simulink model "Position_and_Velocity_Kinematics"  (R2020b)
settings: Solver=VariableStepAuto  StartTime=0.0  StopTime=3  RelTol=1e-3
libraries: simulink x2
settings Model: Creator=barak  LastModifiedBy=barak

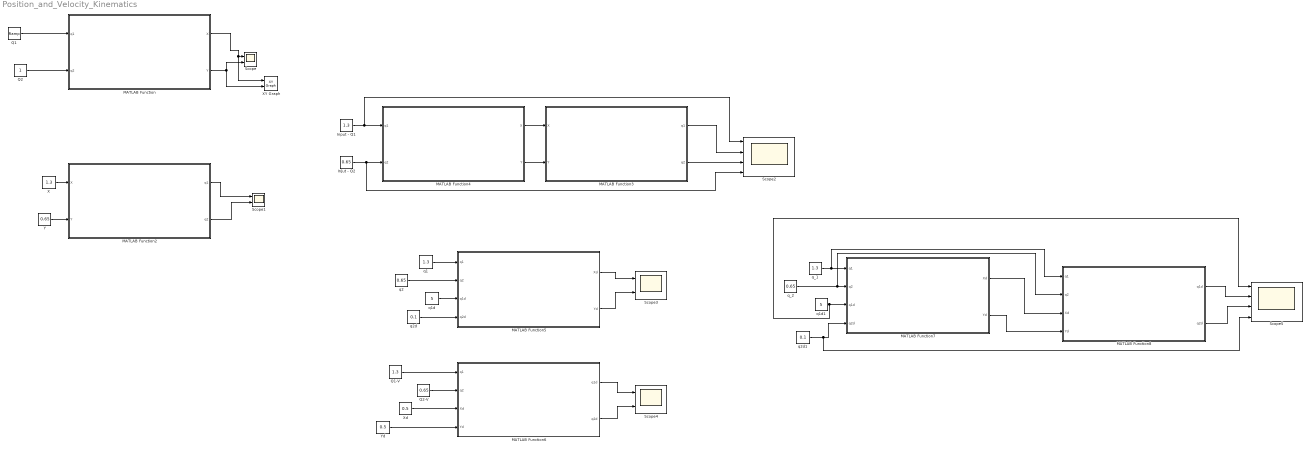
== system Position_and_Velocity_Kinematics ==
  In[ut - Q2 : Constant  Value=0.65
  Input - Q1 : Constant  Value=1.3
  MATLAB Function : MATLAB Function  TreatAsAtomicUnit=on
  MATLAB Function2 : MATLAB Function  TreatAsAtomicUnit=on
  MATLAB Function3 : MATLAB Function  TreatAsAtomicUnit=on
  MATLAB Function4 : MATLAB Function  TreatAsAtomicUnit=on
  MATLAB Function5 : MATLAB Function  TreatAsAtomicUnit=on
  MATLAB Function6 : MATLAB Function  TreatAsAtomicUnit=on
  MATLAB Function7 : MATLAB Function  TreatAsAtomicUnit=on
  MATLAB Function8 : MATLAB Function  TreatAsAtomicUnit=on
  Q1 : simulink/Sources/Ramp  slope=1  start=0  InitialOutput=0
  Q1-V : Constant  Value=1.3
  Q2 : Constant
  Q2-V : Constant  Value=0.65
  Scope{,1,3..4} (4 alike) : Scope  NumInputPorts=2
  Scope2 : Scope  NumInputPorts=4
  Scope5 : Scope  NumInputPorts=4
  X : Constant  Value=1.3
  XY Graph : simulink/Sinks/XY Graph  xmin=-2  xmax=2  ymin=0  ymax=2  st=-1
  Xd : Constant  Value=0.5
  Y : Constant  Value=0.65
  Yd : Constant  Value=0.5
  q1 : Constant  Value=1.3
  q1d : Constant  Value=5
  q1d1 : Constant  Value=5
  q2 : Constant  Value=0.65
  q2d : Constant  Value=0.1
  q2d1 : Constant  Value=0.1
  q_1 : Constant  Value=1.3
  q_2 : Constant  Value=0.65
  wires:
  Q1/1 -> MATLAB Function/1(q1)
  Q2/1 -> MATLAB Function/2(q2)
  MATLAB Function/1(X) -> XY Graph/1, Scope/1
  MATLAB Function/2(Y) -> XY Graph/2, Scope/2
  Y/1 -> MATLAB Function2/2(Y)
  X/1 -> MATLAB Function2/1(X)
  MATLAB Function2/2(q2) -> Scope1/2
  MATLAB Function2/1(q1) -> Scope1/1
  MATLAB Function4/1(X) -> MATLAB Function3/1(X)
  MATLAB Function4/2(Y) -> MATLAB Function3/2(Y)
  In[ut - Q2/1 -> Scope2/4, MATLAB Function4/2(q2)
  Input - Q1/1 -> Scope2/1, MATLAB Function4/1(q1)
  MATLAB Function3/1(q1) -> Scope2/2
  MATLAB Function3/2(q2) -> Scope2/3
  q2/1 -> MATLAB Function5/2(q2)
  q1/1 -> MATLAB Function5/1(q1)
  q1d/1 -> MATLAB Function5/3(q1d)
  q2d/1 -> MATLAB Function5/4(q2d)
  MATLAB Function5/1(Xd) -> Scope3/1
  MATLAB Function5/2(Yd) -> Scope3/2
  Q1-V/1 -> MATLAB Function6/1(q1)
  Q2-V/1 -> MATLAB Function6/2(q2)
  Xd/1 -> MATLAB Function6/3(Xd)
  Yd/1 -> MATLAB Function6/4(Yd)
  MATLAB Function6/2(q2d) -> Scope4/2
  MATLAB Function6/1(q1d) -> Scope4/1
  q2d1/1 -> Scope5/4, MATLAB Function7/4(q2d)
  q_2/1 -> MATLAB Function8/2(q2), MATLAB Function7/2(q2)
  q1d1/1 -> MATLAB Function7/3(q1d), Scope5/1
  q_1/1 -> MATLAB Function8/1(q1), MATLAB Function7/1(q1)
  MATLAB Function7/1(Xd) -> MATLAB Function8/3(Xd)
  MATLAB Function7/2(Yd) -> MATLAB Function8/4(Yd)
  MATLAB Function8/1(q1d) -> Scope5/2
  MATLAB Function8/2(q2d) -> Scope5/3

== matlab function Position_and_Velocity_Kinematics/MATLAB Function ==
  data: q1 input; q2 input; X output; Y output
function [X,Y] = RP_POSITION_FW(q1,q2)
L1 = 0.5;
X = (L1+q2) * cosd(q1);
Y = (L1+q2) * sind(q1);
end

== matlab function Position_and_Velocity_Kinematics/MATLAB Function2 ==
  data: X input; Y input; q1 output; q2 output
function [q1,q2] = RP_POSITION_INV(X,Y)
L1 = 0.5;
q1 = atand(Y/X);
q2 = sqrt(X^2 + Y^2) - L1;
end

== matlab function Position_and_Velocity_Kinematics/MATLAB Function3 ==
  data: X input; Y input; q1 output; q2 output
function [q1,q2] = RP_POSITION_INV(X,Y)
L1 = 0.5;
q1 = atand(Y/X);
q2 = sqrt(X^2 + Y^2) - L1;
end

== matlab function Position_and_Velocity_Kinematics/MATLAB Function4 ==
  data: q1 input; q2 input; X output; Y output
function [X,Y] = RP_POSITION_FW(q1,q2)
L1 = 0.5;
X = (L1+q2) * cosd(q1);
Y = (L1+q2) * sind(q1);
end

== matlab function Position_and_Velocity_Kinematics/MATLAB Function5 ==
  data: q1 input; q2 input; Xd output; Yd output; q1d input; q2d input
function [Xd,Yd] = RP_VELOCITY_FW(q1,q2,q1d,q2d)
L1 = 0.5;
Xd = -(L1+q2) * sind(q1)*q1d + cosd(q1)*q2d;
Yd = (L1+q2) * cosd(q1)*q1d + sind(q1)*q2d;
end

== matlab function Position_and_Velocity_Kinematics/MATLAB Function6 ==
  data: q1 input; q2 input; Xd input; q1d output; Yd input; q2d output
function [q1d,q2d] = RP_VELOCITY_INV(q1,q2,Xd,Yd)
L1=0.5;
J = [-(L1+q2)*sind(q1),cosd(q1);
      (L1+q2)*cosd(q1),sind(q1)];
  Joint_Vel = (J\[Xd;Yd]);
  q1d = Joint_Vel(1);
  q2d = Joint_Vel(2);
end

== matlab function Position_and_Velocity_Kinematics/MATLAB Function7 ==
  data: q1 input; q2 input; Xd output; Yd output; q1d input; q2d input
function [Xd,Yd] = RP_VELOCITY_FW(q1,q2,q1d,q2d)
L1 = 0.5;
Xd = -(L1+q2) * sind(q1)*q1d + cosd(q1)*q2d;
Yd = (L1+q2) * cosd(q1)*q1d + sind(q1)*q2d;
end

== matlab function Position_and_Velocity_Kinematics/MATLAB Function8 ==
  data: q1 input; q2 input; Xd input; q1d output; Yd input; q2d output
function [q1d,q2d] = RP_VELOCITY_INV(q1,q2,Xd,Yd)
L1=0.5;
J = [-(L1+q2)*sind(q1),cosd(q1);
      (L1+q2)*cosd(q1),sind(q1)];
  Joint_Vel = (J\[Xd;Yd]);
  q1d = Joint_Vel(1);
  q2d = Joint_Vel(2);
end
